simulink model "PID1_kalman"  (Simulink 8.5)
settings: Solver=ode45  StartTime=0.0  StopTime=10  RelTol=1e-3
values from neighbouring files (symbols this model uses):
  arm_home = [ -0.1106   -1.9490   -0.1920    3.1840 ]    [NEW_PID_4DOF.m]    (also in SetPoint_Control.m = [ -0.1106   -1.9490   -0.1920    3.1840    0.2825    0.0969 ; Stochastic_coriolis.m = [  -0.1106   -1.9490   -0.1920    3.1840    0.2825    0.0969; Untitled4.m = [ -0.1106   -1.9490   -0.1920    3.1840    0.2825    0.0969 )
undefined symbols (not defined in the file or in its folder): arm_j2mt, arm_m2jp, bit, CAN_init, enc_per_rev, FT_init, get, hot, MT_init, puck_I_per_Nm, sample_time, Standard, VL1_init, VL2_init
libraries: slrtlib x11, simulink x8, slrtsoftinglib x7, dspadpt3 x7, xpcutilitieslib x4, dspsnks4 x1
settings Model: xpc_rtwmakecfg_data=_xpccanac2pci_  Creator=paulghanem  LastModifiedBy=User  SimulationMode=external  ExtModeTrigDuration=50000
settings SolverCC: EnableConcurrentExecution=on
settings DataIOCC: LimitDataPoints=off  MaxDataPoints=5000000  SaveFormat=Dataset  SignalLoggingSaveFormat=Dataset  SaveOutput=off  InspectSignalLogs=on  SaveTime=off  ReturnWorkspaceOutputs=on
settings OptimizationCC: BlockReduction=off  OptimizeBlockIOStorage=off  BufferReuse=off  GlobalBufferReuse=off  ExpressionFolding=off  ExpressionDepthLimit=128  LocalBlockOutputs=off
settings DebuggingCC: UnderspecifiedInitializationDetection=Simplified  MergeDetectMultiDrivingBlocksExec=error  FcnCallInpInsideContextMsg=EnableAllAsError  StateNameClashWarn=none
settings HardwareCC: ProdIntDivRoundTo=Zero  ProdEndianess=LittleEndian  ProdLongLongMode=on  ProdHWDeviceType=Generic->32-bit x86 compatible
settings RTWCC: SystemTargetFile=slrt.tlc  TemplateMakefile=slrt_default_tmf  Description=Simulink Real-Time  RTWVerbose=off
settings SimulinkRealTimeCC: xPCisModelTimeout=off  xPCModelTimeoutSecs=15
settings ConfigComp: CovMetricSettings=dw  CovHtmlReporting=on  CovSaveCumulativeToWorkspaceVar=on  CovSaveSingleToWorkspaceVar=on  CovExternalEMLEnable=off

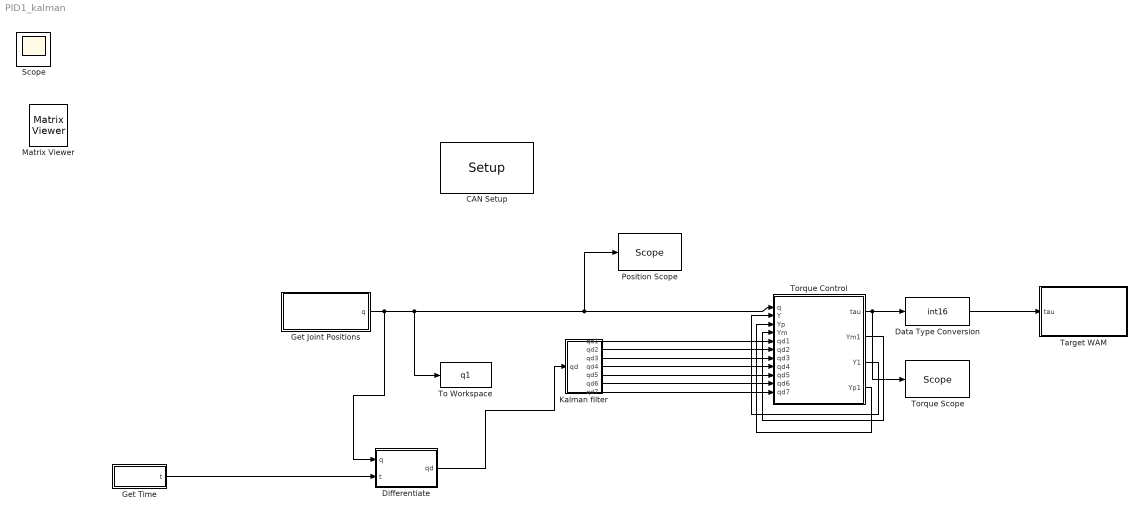
== system PID1_kalman ==
  "CAN Setup " : slrtsoftinglib/CAN-AC2-PCI SJA 1000/Setup   board=1  can1bus=Highspeed (ISO 11898)  can1Baudrate=1 MBaud  can1UserBR=[1,1,4,3]  can2bus=Highspeed (ISO 11898)  can2Baudrate=1 MBaud  can2UserBR=[1,1,4,3]  init=[VL1_init,VL2_init,CAN_init,FT_init,MT_init]  term=[]  bus_off_out=off  bus_off_rec=Off  ioBaseAddress=-1
  Data Type Conversion : DataTypeConversion  OutDataTypeStr=int16
  Differentiate : Subsystem
  Get Joint Positions : Subsystem
  Get Time : Subsystem
  Kalman filter : Subsystem
  Position Scope : slrtlib/Displays and Logging/Scope   scopeno=2  scopetype=Target  autostart=on  viewmode=Numerical  formatstr=['joint_1 %13.8f rad,joint_2 %13.8f rad,joint_3 %13.8f rad,joint_4 %13.8f rad,joint_5 %13.8f rad,joint_6 %13.8f rad,joint_7 %13.8f rad']  grid=on  ylimits=[0,0]  nosamples=1/(10*sample_time)  noprepostsamples=0  interleave=1  triggermode=FreeRun  triggersignal=1  trigsignalfromport=off  triggerlevel=0.0  triggerslope=Either  triggerscope=1  triggersample=0  filename=data.dat  mode=Lazy  writesize=512  autorestart=off  dynamicfilemode=off  maxwritefilesize=512*1024^2
  Target WAM : Subsystem
  To Workspace : ToWorkspace  VariableName=q1  SaveFormat=Structure With Time  SampleTime=-1
  Torque Control : Subsystem
  Torque Scope : slrtlib/Displays and Logging/Scope   scopeno=1  scopetype=Target  autostart=on  viewmode=Numerical  formatstr=['joint_1 %10.5f N-m,joint_2 %10.5f N-m,joint_3 %10.5f N-m,joint_4 %10.5f N-m,joint_5 %10.5f N-m,joint_6 %10.5f N-m,joint_7 %10.5f N-m']  grid=on  ylimits=[0,0]  nosamples=1/(10*sample_time)  noprepostsamples=0  interleave=1  triggermode=FreeRun  triggersignal=1  trigsignalfromport=off  triggerlevel=0.0  triggerslope=Either  triggerscope=1  triggersample=0  filename=data.dat  mode=Lazy  writesize=512  autorestart=off  dynamicfilemode=off  maxwritefilesize=512*1024^2
  Matrix Viewer : dspsnks4/Matrix Viewer  IOType=viewer  ImageParams=off  CMapStr=hot(256)  AxisColorbar=on  AxisParams=off  AxisOrigin=Upper left corner  XLabel=X-axis  YLabel=Y-axis  ZLabel=Z-axis  FigPos=get(0,'defaultfigureposition')  AxisZoom=off
      settings: YMin=-2  YMax=0
  Scope : Scope
  wires:
  Torque Control/1(tau) -> Data Type Conversion/1, Torque Scope/1
  Get Joint Positions/1(q) -> Differentiate/1(q), To Workspace/1, Torque Control/1(q), Position Scope/1
  Data Type Conversion/1 -> Target WAM/1(tau)
  Torque Control/2(Ym1) -> Torque Control/4(Ym)
  Torque Control/3(Y1) -> Torque Control/2(Y)
  Torque Control/4(Yp1) -> Torque Control/3(Yp)
  Differentiate/1(qd) -> Kalman filter/1(qd)
  Get Time/1(t) -> Differentiate/2(t)
  Kalman filter/1(qd1) -> Torque Control/5(qd1)
  Kalman filter/2(qd2) -> Torque Control/6(qd2)
  Kalman filter/3(qd3) -> Torque Control/7(qd3)
  Kalman filter/4(qd4) -> Torque Control/8(qd4)
  Kalman filter/5(qd5) -> Torque Control/9(qd5)
  Kalman filter/6(qd6) -> Torque Control/10(qd6)
  Kalman filter/7(qd7) -> Torque Control/11(qd7)

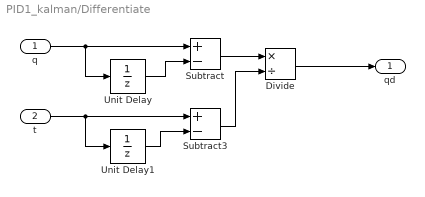
== system PID1_kalman/Differentiate ==
  q : Inport
  t : Inport  Port=2
  Divide : Product  Inputs=*/
  Subtract : Sum  Inputs=+-
  Subtract3 : Sum  Inputs=+-
  Unit Delay : UnitDelay  SampleTime=-1
  Unit Delay1 : UnitDelay  SampleTime=-1
  qd : Outport
  wires:
  q/1 -> Subtract/1, Unit Delay/1
  t/1 -> Unit Delay1/1, Subtract3/1
  Unit Delay1/1 -> Subtract3/2
  Unit Delay/1 -> Subtract/2
  Subtract/1 -> Divide/1
  Divide/1 -> qd/1
  Subtract3/1 -> Divide/2

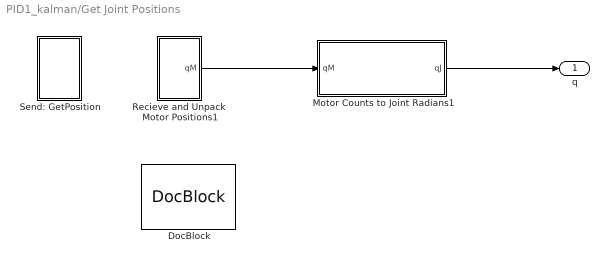
== system PID1_kalman/Get Joint Positions ==
  DocBlock : simulink/Model-Wide Utilities/DocBlock  DocumentType=Text
  Motor Counts to Joint Radians1 : Subsystem
  Recieve and Unpack  Motor Positions1 : Subsystem
  Send: GetPosition : Subsystem
  q : Outport
  wires:
  Motor Counts to Joint Radians1/1(qJ) -> q/1
  Recieve and Unpack  Motor Positions1/1(qM) -> Motor Counts to Joint Radians1/1(qM)

== system PID1_kalman/Get Time ==
  Clock Frequency : Constant  Value=1.193e6
  Divide1 : Product  Inputs=*/
  "xPC Target  Time " : slrtlib/Target Management/Target Information/Session Time   ts=sample_time
  t : Outport
  wires:
  "xPC Target  Time "/1 -> Divide1/1
  Clock Frequency/1 -> Divide1/2
  Divide1/1 -> t/1

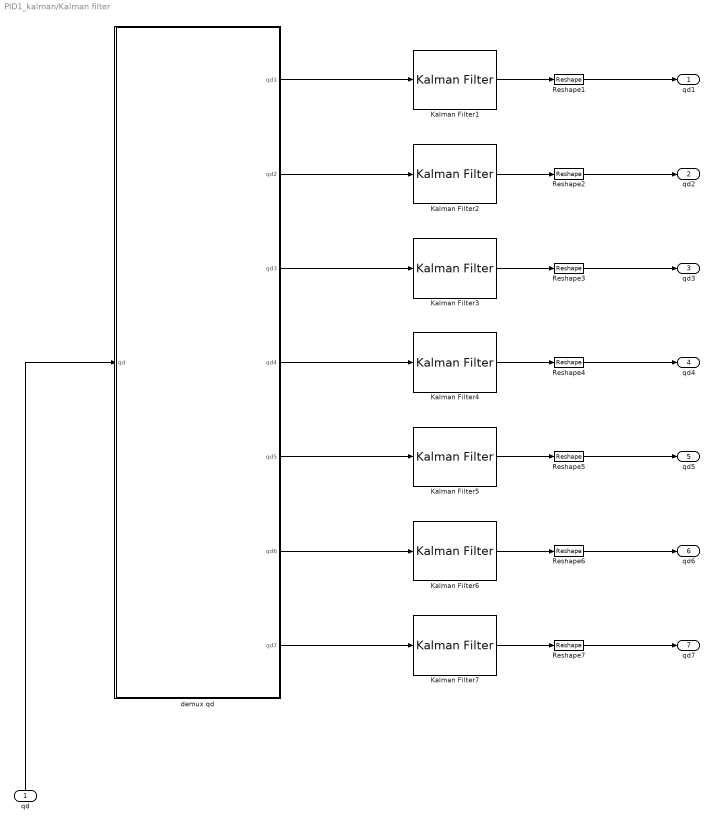
== system PID1_kalman/Kalman filter ==
  qd : Inport
  Kalman Filter1 : dspadpt3/Kalman Filter  num_targets=1  sourceEnable=Always  isReset=off  X=[-0.1106; 0]  P=[1e-4 0 ; 0 1]  A=[1 0.002 ; 0 1]  sourceMeasure=Specify via Dialog  H=[1 0]  Q=[0 0.000 ;0.000 0.004]  R=1e-3  isOutputEstMeasure=on  isOutputEstState=off  isOutputEstError=off  isOutputPrdMeasure=off  isOutputPrdState=off  isOutputPrdError=off
  Kalman Filter2 : dspadpt3/Kalman Filter  num_targets=1  sourceEnable=Always  isReset=on  X=[-1.94900000000000; 0]  P=[1e-4 0 ; 0 1]  A=[1 0.002 ; 0 1]  sourceMeasure=Specify via Dialog  H=[1 0]  Q=[0 0; 0 0.004]  R=5e-2  isOutputEstMeasure=on  isOutputEstState=off  isOutputEstError=off  isOutputPrdMeasure=off  isOutputPrdState=off  isOutputPrdError=off
  Kalman Filter3 : dspadpt3/Kalman Filter  num_targets=1  sourceEnable=Always  isReset=on  X=[-0.192000000000000; 0]  P=[1e-4 0 ; 0 1]  A=[1 0.002 ; 0 1]  sourceMeasure=Specify via Dialog  H=[1 0]  Q=[0 0; 0 0.004]  R=1e-3  isOutputEstMeasure=on  isOutputEstState=off  isOutputEstError=off  isOutputPrdMeasure=off  isOutputPrdState=off  isOutputPrdError=off
  Kalman Filter4 : dspadpt3/Kalman Filter  num_targets=1  sourceEnable=Always  isReset=on  X=[3.18400000000000; 0]  P=[1e-4 0 ; 0 1]  A=[1 0.002 ; 0 1]  sourceMeasure=Specify via Dialog  H=[1 0]  Q=[0 0; 0 0.004]  R=1e-3  isOutputEstMeasure=on  isOutputEstState=off  isOutputEstError=off  isOutputPrdMeasure=off  isOutputPrdState=off  isOutputPrdError=off
  Kalman Filter5 : dspadpt3/Kalman Filter  num_targets=1  sourceEnable=Always  isReset=on  X=[0.282500000000000; 0]  P=[1e-4 0 ; 0 1]  A=[1 0.002 ; 0 1]  sourceMeasure=Specify via Dialog  H=[1 0]  Q=[0 0; 0 0.004]  R=1e-6  isOutputEstMeasure=on  isOutputEstState=off  isOutputEstError=off  isOutputPrdMeasure=off  isOutputPrdState=off  isOutputPrdError=off
  Kalman Filter6 : dspadpt3/Kalman Filter  num_targets=1  sourceEnable=Always  isReset=on  X=[0.0969000000000000; 0]  P=[1e-4 0 ; 0 1]  A=[1 0.002 ; 0 1]  sourceMeasure=Specify via Dialog  H=[1 0]  Q=[0 0; 0 0.004]  R=1e-6  isOutputEstMeasure=on  isOutputEstState=off  isOutputEstError=off  isOutputPrdMeasure=off  isOutputPrdState=off  isOutputPrdError=off
  Kalman Filter7 : dspadpt3/Kalman Filter  num_targets=1  sourceEnable=Always  isReset=on  X=[-0.279800000000000; 0]  P=[1e-4 0 ; 0 1]  A=[1 0.002 ; 0 1]  sourceMeasure=Specify via Dialog  H=[1 0]  Q=[0 0; 0 0.004]  R=1e-6  isOutputEstMeasure=on  isOutputEstState=off  isOutputEstError=off  isOutputPrdMeasure=off  isOutputPrdState=off  isOutputPrdError=off
  Reshape{1..7} (7 alike) : Reshape
  demux qd : Subsystem
  qd1 : Outport
  qd2 : Outport  Port=2
  qd3 : Outport  Port=3
  qd4 : Outport  Port=4
  qd5 : Outport  Port=5
  qd6 : Outport  Port=6
  qd7 : Outport  Port=7
  wires:
  Reshape7/1 -> qd7/1
  Kalman Filter7/1 -> Reshape7/1
  qd/1 -> demux qd/1(qd)
  demux qd/7(qd7) -> Kalman Filter7/1
  demux qd/4(qd4) -> Kalman Filter4/1
  Kalman Filter5/1 -> Reshape5/1
  Reshape5/1 -> qd5/1
  demux qd/5(qd5) -> Kalman Filter5/1
  demux qd/2(qd2) -> Kalman Filter2/1
  demux qd/3(qd3) -> Kalman Filter3/1
  Kalman Filter3/1 -> Reshape3/1
  Kalman Filter2/1 -> Reshape2/1
  Reshape3/1 -> qd3/1
  Reshape2/1 -> qd2/1
  demux qd/6(qd6) -> Kalman Filter6/1
  Reshape6/1 -> qd6/1
  Kalman Filter6/1 -> Reshape6/1
  Kalman Filter4/1 -> Reshape4/1
  Reshape4/1 -> qd4/1
  Reshape1/1 -> qd1/1
  Kalman Filter1/1 -> Reshape1/1
  demux qd/1(qd1) -> Kalman Filter1/1

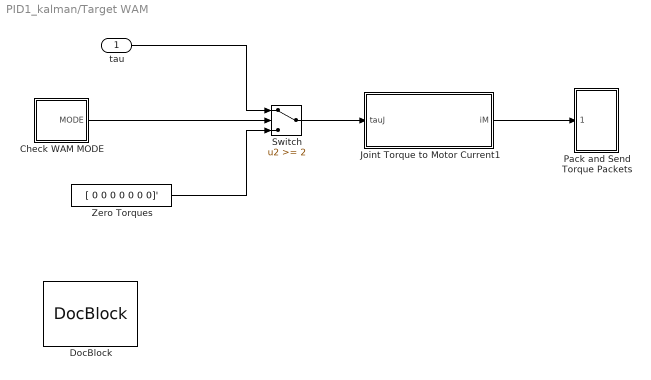
== system PID1_kalman/Target WAM ==
  tau : Inport
  Check WAM MODE : Subsystem
  DocBlock : simulink/Model-Wide Utilities/DocBlock  DocumentType=Text
      content=|
      | This block does all of the communication with the WAM over the CAN card.
      | First we check the WAM mode to see if it in is Shift-Idle or Shift-Active
      | mode. It is necessary to pass this as output, so that PID knows whether it
      | should be integrating on the error or not. If we are in Shift-Idle mode,
      | we send zero torques. Also in this block, we convert joint torque to motor
      | current using the transformations in the documentation. Then we pack the
      | torque packets into a CAN message and send it.
      |
      | To receive joint positions we also send a CAN message which will respond
      | back with the appropriate information. Once we receive the joint positions,
      | we need to differentiate it to get joint velocities (since the WAM does not
      | have tachometers). Finally, passing it through a moving average of the last
      | n readings removes some of the noise and gives us a smoother velocity
      | signal.
  Joint Torque to Motor Current1 : Subsystem
  Pack and Send Torque Packets : Subsystem
  Switch : Switch  Threshold=2
  Zero Torques : Constant  Value=[ 0 0 0 0 0 0 0]'  OutDataTypeStr=int16
  wires:
  Joint Torque to Motor Current1/1(iM) -> Pack and Send Torque Packets/1(Current)
  Switch/1 -> Joint Torque to Motor Current1/1(tauJ)
  tau/1 -> Switch/1
  Zero Torques/1 -> Switch/3
  Check WAM MODE/1(MODE) -> Switch/2

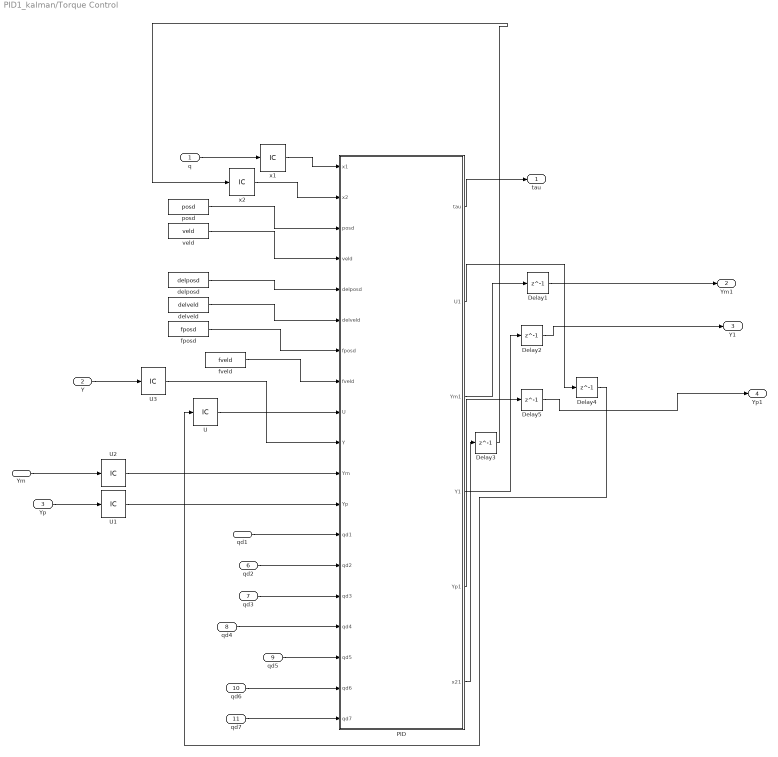
== system PID1_kalman/Torque Control ==
  q : Inport
  Y : Inport  Port=2  PortDimensions=[14]
  Yp : Inport  Port=3  PortDimensions=[14]
  Ym : Inport  Port=4  PortDimensions=[14]
  qd1 : Inport  Port=5
  qd2 : Inport  Port=6
  qd3 : Inport  Port=7
  qd4 : Inport  Port=8
  qd5 : Inport  Port=9
  qd6 : Inport  Port=10
  qd7 : Inport  Port=11
  Delay{1..5} (5 alike) : Delay  DelayLength=1  InitialCondition=0
  PID : MATLAB Function  TreatAsAtomicUnit=on
  U : InitialCondition  Value=[0 0 0 0 0 0 0]
  U1 : InitialCondition  Value="[-0.118379466216232\t-1.94549765955054\t-0.0293926790562203\t3.12033974637458\t0.240671515435818\t-0.0680676596254651\t-0.117976842537181 0 0 0 0 0 0 0]"
  U2 : InitialCondition  Value="[-0.118379466216232\t-1.94549765955054\t-0.0293926790562203\t3.12033974637458\t0.240671515435818\t-0.0680676596254651\t-0.117976842537181 0 0 0 0 0 0 0]"
  U3 : InitialCondition  Value=[-0.118379466216232 -1.94549765955054 -0.0293926790562203 3.12033974637458 0.240671515435818 -0.068067659625465 -0.117976842537181 0 0 0 0 0 0 0]
  "delposd " : FromWorkspace  VariableName=delposd  SampleTime=sample_time
  delveld : FromWorkspace  VariableName=delveld  SampleTime=sample_time
  "fposd " : FromWorkspace  VariableName=fposd  SampleTime=sample_time
  fveld : FromWorkspace  VariableName=fveld  SampleTime=sample_time
  "posd " : FromWorkspace  VariableName=posd  SampleTime=sample_time
  veld : FromWorkspace  VariableName=veld  SampleTime=sample_time
  x1 : InitialCondition  Value="[-0.118379466216232\t-1.94549765955054\t-0.0293926790562203\t3.12033974637458\t0.240671515435818\t-0.0680676596254651\t-0.117976842537181]"
  x2 : InitialCondition  Value=[0 0 0 0 0 0 0]
  tau : Outport
  Ym1 : Outport  Port=2  PortDimensions=[14]
  Y1 : Outport  Port=3  PortDimensions=[14]
  Yp1 : Outport  Port=4  PortDimensions=[14]
  wires:
  PID/1(tau) -> tau/1
  q/1 -> x1/1
  x1/1 -> PID/1(x1)
  PID/6(x21) -> Delay3/1
  Delay3/1 -> x2/1
  PID/2(U1) -> Delay4/1
  Delay4/1 -> U/1
  U/1 -> PID/9(U)
  x2/1 -> PID/2(x2)
  "posd "/1 -> PID/3(posd)
  veld/1 -> PID/4(veld)
  "delposd "/1 -> PID/5(delposd)
  delveld/1 -> PID/6(delveld)
  "fposd "/1 -> PID/7(fposd)
  fveld/1 -> PID/8(fveld)
  PID/3(Ym1) -> Delay1/1
  PID/4(Y1) -> Delay2/1
  PID/5(Yp1) -> Delay5/1
  Delay1/1 -> Ym1/1
  Delay2/1 -> Y1/1
  Delay5/1 -> Yp1/1
  Y/1 -> U3/1
  Ym/1 -> U2/1
  Yp/1 -> U1/1
  U3/1 -> PID/10(Y)
  U2/1 -> PID/11(Ym)
  U1/1 -> PID/12(Yp)
  qd1/1 -> PID/13(qd1)
  qd3/1 -> PID/15(qd3)
  qd5/1 -> PID/17(qd5)
  qd2/1 -> PID/14(qd2)
  qd4/1 -> PID/16(qd4)
  qd6/1 -> PID/18(qd6)
  qd7/1 -> PID/19(qd7)

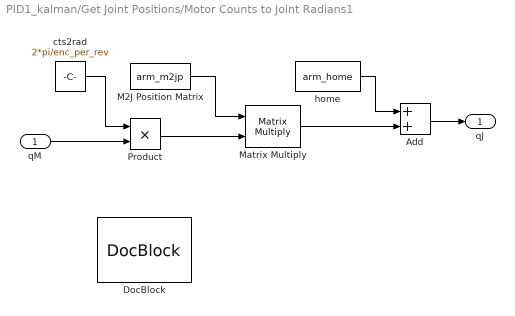
== system PID1_kalman/Get Joint Positions/Motor Counts to Joint Radians1 ==
  qM : Inport
  Add : Sum
  DocBlock : simulink/Model-Wide Utilities/DocBlock  DocumentType=Text
      content=|
      | Here we do the simple conversion from motor position to joint position,
      | then convert encoder counts to joint radians, then account for the offset
      | in the home position to finally output the joint position in radians. The
      | M2J position matrix can be found in the documentation. Joint 4 has a -18 as
      | opposed to +18 because the motor was reversed at one point during a repair.
      | I believe newer models of the WAM adhere to this -18.
  M2J Position Matrix : Constant  Value=arm_m2jp
  Matrix Multiply : Product  Multiplication=Matrix(*)
  Product : Product  OutMin=[-8192]  OutMax=[8191]  RndMeth=Zero
  cts2rad : Constant  Value=2*pi/enc_per_rev
  home : Constant  Value=arm_home
  qJ : Outport
  wires:
  qM/1 -> Product/2
  Add/1 -> qJ/1
  Matrix Multiply/1 -> Add/2
  home/1 -> Add/1
  cts2rad/1 -> Product/1
  M2J Position Matrix/1 -> Matrix Multiply/1
  Product/1 -> Matrix Multiply/2

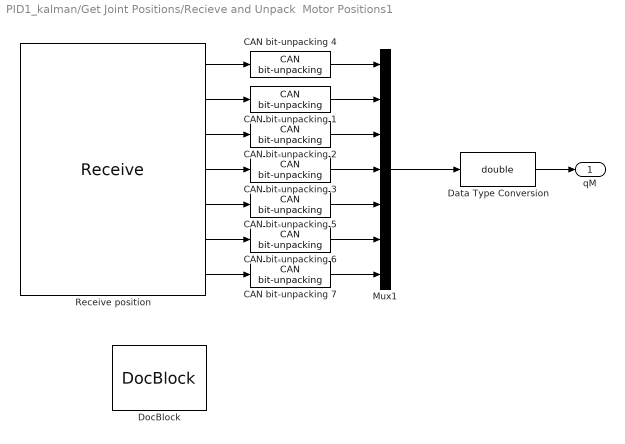
== system PID1_kalman/Get Joint Positions/Recieve and Unpack  Motor Positions1 ==
  CAN bit-unpacking {1..7} (7 alike) : slrtlib/CAN/Utilities/CAN bit-unpacking   bitpatterns={ [16:23, 8:15, 0:5,-1, -1] }  dtypes={ 'int32'}
  Data Type Conversion : DataTypeConversion  OutDataTypeStr=double
  DocBlock : simulink/Model-Wide Utilities/DocBlock  DocumentType=Text
  Mux1 : Mux  Inputs=7
  "Receive position " : slrtsoftinglib/CAN-AC2-PCI SJA 1000/Receive   board=1  canPort=CAN 1  range=Standard (11-bit)  ids=[bin2dec('10000100011'),bin2dec('10001000011'),bin2dec('10001100011'),bin2dec('10010000011'),bin2dec('10010100011'),bin2dec('10011000011'),bin2dec('10011100011')]  lengths=0  output=Data  inten=on  ts=sample_time  ididx=[0,1,2,3,5,6,7]
  qM : Outport
  wires:
  Mux1/1 -> Data Type Conversion/1
  "Receive position "/1 -> CAN bit-unpacking 4/1
  "Receive position "/2 -> CAN bit-unpacking 1/1
  "Receive position "/3 -> CAN bit-unpacking 2/1
  "Receive position "/4 -> CAN bit-unpacking 3/1
  CAN bit-unpacking 4/1 -> Mux1/1
  CAN bit-unpacking 1/1 -> Mux1/2
  CAN bit-unpacking 2/1 -> Mux1/3
  CAN bit-unpacking 3/1 -> Mux1/4
  Data Type Conversion/1 -> qM/1
  "Receive position "/5 -> CAN bit-unpacking 5/1
  "Receive position "/6 -> CAN bit-unpacking 6/1
  "Receive position "/7 -> CAN bit-unpacking 7/1
  CAN bit-unpacking 5/1 -> Mux1/5
  CAN bit-unpacking 6/1 -> Mux1/6
  CAN bit-unpacking 7/1 -> Mux1/7

== system PID1_kalman/Get Joint Positions/Send: GetPosition ==
  Bit Packing : xpcutilitieslib/Bit Packing   MaskBitPatterns={[0:7]}  MaskPackDataType=double  MaskPackDataSize=[1]
  DocBlock : simulink/Model-Wide Utilities/DocBlock  DocumentType=Text
  Send to all motors : slrtsoftinglib/CAN-AC2-PCI SJA 1000/Send   board=1  canPort=CAN 1  range=Standard (11-bit)  ids=1024  sizes=[1]  output=off  ts=sample_time  ididx=[2]
  get position : Constant  Value=[48]  OutDataTypeStr=int8
  wires:
  Bit Packing/1 -> Send to all motors/1
  get position/1 -> Bit Packing/1

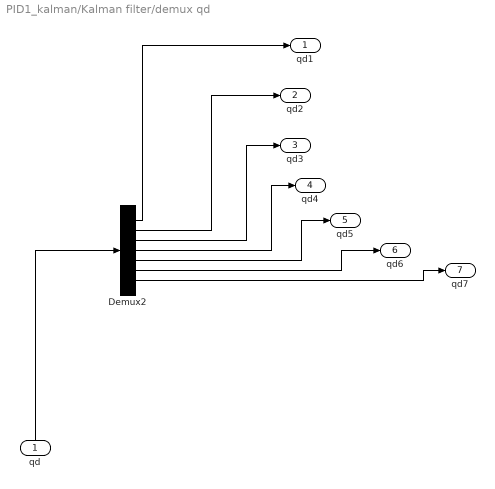
== system PID1_kalman/Kalman filter/demux qd ==
  qd : Inport
  Demux2 : Demux  Outputs=7
  qd1 : Outport
  qd2 : Outport  Port=2
  qd3 : Outport  Port=3
  qd4 : Outport  Port=4
  qd5 : Outport  Port=5
  qd6 : Outport  Port=6
  qd7 : Outport  Port=7
  wires:
  qd/1 -> Demux2/1
  Demux2/1 -> qd1/1
  Demux2/2 -> qd2/1
  Demux2/3 -> qd3/1
  Demux2/4 -> qd4/1
  Demux2/5 -> qd5/1
  Demux2/6 -> qd6/1
  Demux2/7 -> qd7/1

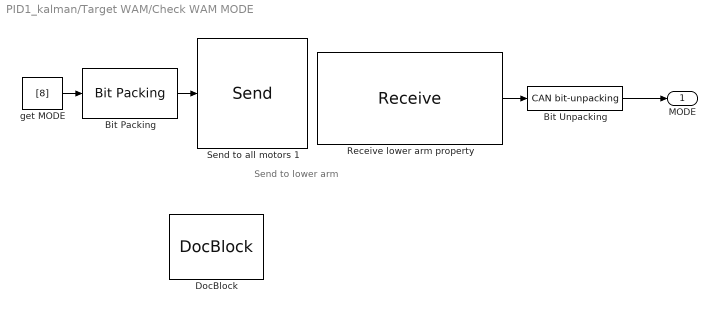
== system PID1_kalman/Target WAM/Check WAM MODE ==
  note: Send to lower arm
  "Bit Packing " : xpcutilitieslib/Bit Packing   MaskBitPatterns={[0:7]}  MaskPackDataType=double  MaskPackDataSize=[1]
  Bit Unpacking : slrtlib/CAN/Utilities/CAN bit-unpacking   bitpatterns={[16:31]}  dtypes={ 'int16'}
  DocBlock : simulink/Model-Wide Utilities/DocBlock  DocumentType=Text
      content=|
      | Here we send an 8 to the lower arm. Property 8 is the MODE and the
      | 1028 (1 00000 00100) means to "set a lower arm property". Finally we
      | receive the mode property from CAN ID 1158, then do some bit unpacking.
      | All of this is well documentated in the "CAN Communication Spec" of the
      | Barrett documentation.
  Receive lower arm property : slrtsoftinglib/CAN-AC2-PCI SJA 1000/Receive   board=1  canPort=CAN 1  range=Standard (11-bit)  ids=[bin2dec('10010000110')]  lengths=0  output=Data  inten=on  ts=sample_time  ididx=[4]
  Send to all motors 1 : slrtsoftinglib/CAN-AC2-PCI SJA 1000/Send   board=1  canPort=CAN 1  range=Standard (11-bit)  ids=[1028]  sizes=[1]  output=off  ts=sample_time  ididx=[5]
  get MODE : Constant  Value=[8]  OutDataTypeStr=uint8
  MODE : Outport
  wires:
  "Bit Packing "/1 -> Send to all motors 1/1
  Receive lower arm property/1 -> Bit Unpacking/1
  get MODE/1 -> "Bit Packing "/1
  Bit Unpacking/1 -> MODE/1

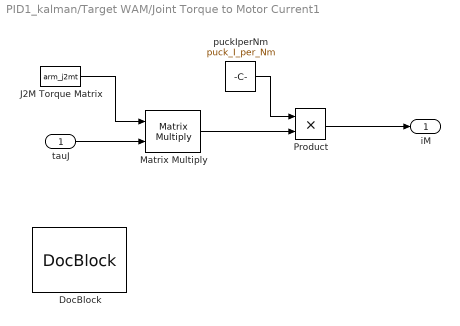
== system PID1_kalman/Target WAM/Joint Torque to Motor Current1 ==
  tauJ : Inport
  DocBlock : simulink/Model-Wide Utilities/DocBlock  DocumentType=Text
  J2M Torque Matrix : Constant  Value=arm_j2mt
  Matrix Multiply : Product  Multiplication=Matrix(*)
  Product : Product  RndMeth=Zero
  puckIperNm : Constant  Value=puck_I_per_Nm
  iM : Outport
  wires:
  J2M Torque Matrix/1 -> Matrix Multiply/1
  Matrix Multiply/1 -> Product/2
  puckIperNm/1 -> Product/1
  Product/1 -> iM/1
  tauJ/1 -> Matrix Multiply/2

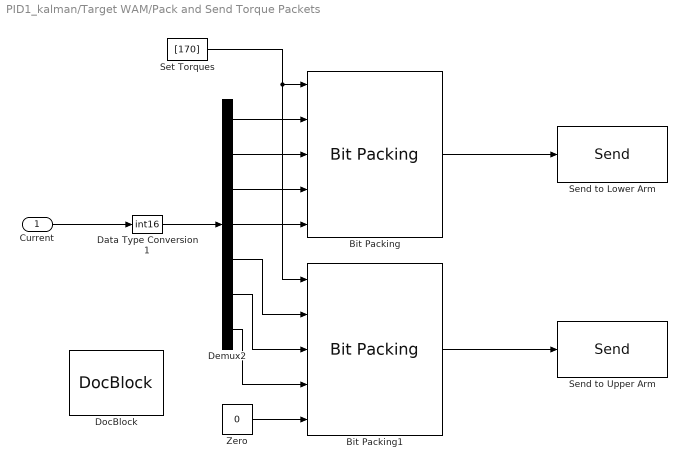
== system PID1_kalman/Target WAM/Pack and Send Torque Packets ==
  Current : Inport
  Bit Packing : xpcutilitieslib/Bit Packing   MaskBitPatterns={[0:7] [18:23 8:15] [36:39 24:31 16:17] [54:55 40:47 32:35] [56:63 48:53]}  MaskPackDataType=double  MaskPackDataSize=[1]
  Bit Packing1 : xpcutilitieslib/Bit Packing   MaskBitPatterns={[0:7] [18:23 8:15] [36:39 24:31 16:17] [54:55 40:47 32:35] [56:63 48:53]}  MaskPackDataType=double  MaskPackDataSize=[1]
  Data Type Conversion1 : DataTypeConversion  OutMin=[-8191]  OutMax=[8191]  OutDataTypeStr=int16  RndMeth=Zero
  Demux2 : Demux  Outputs=7
  DocBlock : simulink/Model-Wide Utilities/DocBlock  DocumentType=Text
  Send to Lower Arm : slrtsoftinglib/CAN-AC2-PCI SJA 1000/Send   board=1  canPort=CAN 1  range=Standard (11-bit)  ids=bin2dec('10000000001')  sizes=[8]  output=off  ts=sample_time  ididx=[3]
  Send to Upper Arm : slrtsoftinglib/CAN-AC2-PCI SJA 1000/Send   board=1  canPort=CAN 1  range=Standard (11-bit)  ids=bin2dec('10000000010')  sizes=[8]  output=off  ts=sample_time  ididx=[4]
  "Set Torques " : Constant  Value=[170]  OutDataTypeStr=uint8
  Zero : Constant  Value=0  OutDataTypeStr=int16
  wires:
  "Set Torques "/1 -> Bit Packing/1, Bit Packing1/1
  Bit Packing/1 -> Send to Lower Arm/1
  Demux2/1 -> Bit Packing/2
  Demux2/2 -> Bit Packing/3
  Demux2/3 -> Bit Packing/4
  Demux2/4 -> Bit Packing/5
  Current/1 -> Data Type Conversion1/1
  Data Type Conversion1/1 -> Demux2/1
  Bit Packing1/1 -> Send to Upper Arm/1
  Demux2/5 -> Bit Packing1/2
  Demux2/6 -> Bit Packing1/3
  Demux2/7 -> Bit Packing1/4
  Zero/1 -> Bit Packing1/5

== matlab function Torque Control/PID ==
  data: x1 input double; x2 input double; posd input double; tau output double; veld input double; delposd input double; delveld input double; fposd input double; fveld input double; U input double; U1 output double; Ym1 output double; Y1 output double; Yp1 output double; x21 output double; Y input double; Ym input double; Yp input double; qd1 input double; qd2 input double; qd3 input double; qd4 input double; qd5 input double; qd6 input double; qd7 input double
%
% gravComp7DOFNum Compute inverse dynamics via recursive Newton-Euler formulation
%
% Recursive Newton-Euler for standard Denavit-Hartenberg notation.
%

% Copyright (C) 1993-2011, by Peter I. Corke
%
% This file originally was part of The Robotics Toolbox for Matlab (RTB).
%
% http://www.petercorke.com

%
% Simplified from rne_dh for 7DOF WAM to compute only torque from gravity by Hans Vorsteveld
% Does not use structures from RTB, only the RNE algorithm
%

function [tau,U1,Ym1,Y1,Yp1,x21] = PID(x1,x2,posd,veld,delposd,delveld,fposd,fveld,U,Y,Ym,Yp,qd1,qd2,qd3,qd4,qd5,qd6,qd7)

%-------------------------------------------------------------------------------------
%   SETUP THE ARM
%-------------------------------------------------------------------------------------    
    n = 14;p = 7; q = 14;
    
 Ts=0.002; 


 


yddel=[delposd;delveld];
yd = [posd;veld];
fyd=[fposd;fveld];


 

%initial conditions
%x1 = [-0.11060;-1.949;-0.1920;3.1840;0.2825;0.09690;-0.27980];
%x2 = zeros(7,1);
%U = zeros(7,1);
Ae = (1-Ts)*eye(n);
C= eye(14);
Ce = C;
Iq = eye(q);
Oq = zeros(q);
H = [Iq Oq Oq -Ce*Ae;Iq Oq Oq zeros(q,n);Oq Iq Oq zeros(q,n);zeros(n,q) zeros(n,q) zeros(n,q) Ae];
Ib = zeros(3*q,3*q+n);
for k11 = 1:3*q,Ib(k11,k11) = 1;end
sig = 1e-4;
sigR = sig;
sigQ = 1e-3;
P = 1e-8*eye(3*q+n);
Rb = (sigR^2)*diag(1*ones(3*q,1));
Q = sigQ^2*eye(n);





 Be = Ts*[zeros(7,7);inv(D(x1))];
    Delyd=[fyd-yd];
    Del2yd = Delyd*Delyd';
   
    Gd = [Del2yd Oq Oq zeros(q,n); Oq Oq Oq zeros(q,n); Oq Oq Oq zeros(q,n);zeros(n,q) zeros(n,q) zeros(n,q) Q];
   
    
    
    EE = [Ce*Be;zeros(q,p);zeros(q,p);-Be];
    K = inv(EE'*EE)*EE'*H*P*Ib'*inv(Ib*P*Ib' + Rb);
    PHI = H - EE*K*Ib;

     P = PHI*P*PHI' + EE*K*Rb*K'*EE' + Gd;
    K1 = K(:,1:q);
    K2 = K(:,q+1:2*q);
    K3 = K(:,2*q+1:3*q);
    
    
      %  E = yd - Y ;
       % Ep = ydfut-Yp ;
        %U = U + K1*Ep + K2*E;
        %Ym = Y;
        %Y = Yp;
         %x_1 = x1 ;
       
         %x_11 = x_1; %Since at t=0, velocity is zero
        %XX2 = zeros(7,1);
        %x_22= (-inv(D(x_1))*(transpose(G(x_1)))+ inv(D(x_1))*U)*Ts + XX2 ;
        %Yp = [x_11' x_22']';
       
    
        Em = yddel - Ym ;
        E = yd - Y ;
        Ep = fyd-Yp ;
        U = U + K1*Ep + K2*E + K3*Em;
        Ym = Y;
        Y = Yp;
        
        x_1 = x1;
        
         %
        pos_meas = x1 ; % In experimental work you do not add noise instead you only use measurement of position
        x_11 =  x2*Ts + pos_meas; % Here we are estimating position using the extimate of x2 and measurement of x1 at present time
        
       % XX2 = (x_11-x_1)/Ts; %
       XX2=[qd1;qd2;qd3;qd4;qd5;qd6;qd7];
       
        x_22= (-inv(D(pos_meas))*((G(pos_meas)))+ inv(D(pos_meas))*U)*Ts + XX2 ;
       
       
        
        Yp = [x_11' x_22']';
        tau=U;
        Yp1=Yp;
        Ym1=Ym;
        Y1=Y;
        U1=U;
        x21= x_22;
    
   
end 

function G = G(q)

DH_a = [0 0 0.045 -0.045 0 0 0];
    DH_d = [0 0 .55 0 0.3 0 0.061];
    DH_alpha = [-pi/2 pi/2 -pi/2 pi/2 -pi/2 pi/2 0];
 
    m = [10.7676 3.87 1.8022 2.4 0.1237 0.4979886 0.07548270];
    
    com = zeros(3,7);
    com(:,1) = [-0.00443422; 0.12189039; -0.00066489];
    com(:,2) = [-0.00236983; 0.03105614; 0.01542114 ];
    com(:,3) = [-0.03825858; 0.20750770; 0.00003309];
    com(:,4) = [ 0.00498512;-0.00022942;0.13271662 ];
    com(:,5) = [0.00008921;0.00511217;0.00435824];
    com(:,6) = [-0.00012262;-0.01703194;0.02468336];
    com(:,7) = [-0.00007974;0.00016313;-0.00323552 ];
     
    
    T = zeros(4,4,7);
     
for j=1:7,
        a = DH_a(j);
        d = DH_d(j);
        alpha = DH_alpha(j);
        T(:,:,j) = getTransformDH(a, d, alpha, q(j));
end 
comstar = zeros(4,7);
    comstar(:,1) = [com(:,1);1];
    comstar(:,2) = [com(:,2);1];
    comstar(:,3) = [com(:,3);1];
    comstar(:,4) = [com(:,4);1];
    comstar(:,5) = [com(:,5);1];
    comstar(:,6) = [com(:,6);1];
    comstar(:,7) = [ com(:,7);1];
  
    Q=[0,-1,0,0;
     1,0,0,0;
     0,0,0,0;
     0,0,0,0];
   
 gravity=[0,0,-9.81,0];
 G=zeros(7,1);
 
   G(1)= -m(1)*gravity*Q*T(:,:,1)*comstar(:,1)-m(2)*gravity*Q*T(:,:,1)*T(:,:,2)*comstar(:,2)-m(3)*gravity*Q*T(:,:,1)*T(:,:,2)*T(:,:,3)*comstar(:,3)-m(4)*gravity*Q*T(:,:,1)*T(:,:,2)*T(:,:,3)*T(:,:,4)*comstar(:,4)-m(5)*gravity*Q*T(:,:,1)*T(:,:,2)*T(:,:,3)*T(:,:,4)*T(:,:,5)*comstar(:,5)-m(6)*gravity*Q*T(:,:,1)*T(:,:,2)*T(:,:,3)*T(:,:,4)*T(:,:,5)*T(:,:,6)*comstar(:,6)-m(7)*gravity*Q*T(:,:,1)*T(:,:,2)*T(:,:,3)*T(:,:,4)*T(:,:,5)*T(:,:,6)*T(:,:,7)*comstar(:,7);   
   G(2)= -m(2)*gravity*T(:,:,1)*Q*T(:,:,2)*comstar(:,2)-m(3)*gravity*T(:,:,1)*Q*T(:,:,2)*T(:,:,3)*comstar(:,3)-m(4)*gravity*T(:,:,1)*Q*T(:,:,2)*T(:,:,3)*T(:,:,4)*comstar(:,4)-m(5)*gravity*T(:,:,1)*Q*T(:,:,2)*T(:,:,3)*T(:,:,4)*T(:,:,5)*comstar(:,5)-m(6)*gravity*T(:,:,1)*Q*T(:,:,2)*T(:,:,3)*T(:,:,4)*T(:,:,5)*T(:,:,6)*comstar(:,6)-m(7)*gravity*T(:,:,1)*Q*T(:,:,2)*T(:,:,3)*T(:,:,4)*T(:,:,5)*T(:,:,6)*T(:,:,7)*comstar(:,7);
   G(3)= -m(3)*gravity*T(:,:,1)*T(:,:,2)*Q*T(:,:,3)*comstar(:,3)-m(4)*gravity*T(:,:,1)*T(:,:,2)*Q*T(:,:,3)*T(:,:,4)*comstar(:,4)-m(5)*gravity*T(:,:,1)*T(:,:,2)*Q*T(:,:,3)*T(:,:,4)*T(:,:,5)*comstar(:,5)-m(6)*gravity*T(:,:,1)*T(:,:,2)*Q*T(:,:,3)*T(:,:,4)*T(:,:,5)*T(:,:,6)*comstar(:,6)-m(7)*gravity*T(:,:,1)*T(:,:,2)*Q*T(:,:,3)*T(:,:,4)*T(:,:,5)*T(:,:,6)*T(:,:,7)*comstar(:,7);
   G(4)= -m(4)*gravity*T(:,:,1)*T(:,:,2)*T(:,:,3)*Q*T(:,:,4)*comstar(:,4)-m(5)*gravity*T(:,:,1)*T(:,:,2)*T(:,:,3)*Q*T(:,:,4)*T(:,:,5)*comstar(:,5)-m(6)*gravity*T(:,:,1)*T(:,:,2)*T(:,:,3)*Q*T(:,:,4)*T(:,:,5)*T(:,:,6)*comstar(:,6)-m(7)*gravity*T(:,:,1)*T(:,:,2)*T(:,:,3)*Q*T(:,:,4)*T(:,:,5)*T(:,:,6)*T(:,:,7)*comstar(:,7);
   G(5)= -m(5)*gravity*T(:,:,1)*T(:,:,2)*T(:,:,3)*T(:,:,4)*Q*T(:,:,5)*comstar(:,5)-m(6)*gravity*T(:,:,1)*T(:,:,2)*T(:,:,3)*T(:,:,4)*Q*T(:,:,5)*T(:,:,6)*comstar(:,6)-m(7)*gravity*T(:,:,1)*T(:,:,2)*T(:,:,3)*T(:,:,4)*Q*T(:,:,5)*T(:,:,6)*T(:,:,7)*comstar(:,7);
   G(6)= -m(6)*gravity*T(:,:,1)*T(:,:,2)*T(:,:,3)*T(:,:,4)*T(:,:,5)*Q*T(:,:,6)*comstar(:,6)-m(7)*gravity*T(:,:,1)*T(:,:,2)*T(:,:,3)*T(:,:,4)*T(:,:,5)*Q*T(:,:,6)*T(:,:,7)*comstar(:,7);
   G(7)= -m(7)*gravity*T(:,:,1)*T(:,:,2)*T(:,:,3)*T(:,:,4)*T(:,:,5)*T(:,:,6)*Q*T(:,:,7)*comstar(:,7);
   
end 
function bq = bq(qd)
 
 
 
s=20;
bc = [2.516; 2.581; 2.038; 0.956; 0.323; 0.315; 0.066];
B =  [1.142; 0.946; 0.309; 0.255; 0.025; 0.039; 0.004];
 
bq = bc.*atan(s*qd)*2/pi+B.*qd;
end 

function D =D(q)
DH_a = [0 0 0.045 -0.045 0 0 0];
    DH_d = [0 0 .55 0 0.3 0 0.061];
    DH_alpha = [-pi/2 pi/2 -pi/2 pi/2 -pi/2 pi/2 0];
 
    m = [10.7676 3.87 1.8022 2.4 0.1237 0.4179886 0.07548270];
    
     
    
    com = zeros(3,7);
   com(:,1) = [-0.00443422; 0.12189039; -0.00066489];
    com(:,2) = [-0.00236983; 0.03105614; 0.01542114 ];
    com(:,3) = [-0.03825858; 0.20750770; 0.00003309];
    com(:,4) = [ 0.00498512;-0.00022942;0.13271662 ];
    com(:,5) = [0.00008921;0.00511217;0.00435824];
    com(:,6) = [-0.00012262;-0.01703194;0.02468336];
    com(:,7) = [-0.00007974;0.00016313;-0.00323552 ];
     
    I=zeros(3,3,7);
    
     I(:,:,1) = [ 0.29486350 , -0.00795023 ,-0.00009311;
                 -0.00795023 , 0.11350017 , -0.00018711;
                -0.00009311 , -0.00018711 , 0.25065343];
    I(:,:,2) =[0.02606840 ,-0.00001346 , -0.00011701;
               -0.00001346,  0.01472202 ,0.00003659;
               -0.00011701 , 0.00003659,  0.01934814];
    I(:,:,3) = [0.13671601,  -0.01680434,  0.00000510;
               -0.01680434 , 0.00588354 , -0.00000530;
                0.00000510 , -0.00000530 , 0.13951371];
    I(:,:,4) = [ 0.05719268 , 0.00001467 , 0.00008193;
                 0.00001467 , 0.05716470 , -0.00009417;
                 0.00008193 , -0.00009417 , 0.00300441] ;
    I(:,:,5) =[0.00005587 , 0.00000026,  0.00000000;
               0.00000026 , 0.00007817,  -0.00000083;
               0.00000000 , -0.00000083,  0.00006594];
    I(:,:,6) = [0.00093106,  0.00000148 , -0.00000201;
                0.00000148,  0.00049833 , -0.00022162;
               -0.00000201,  -0.00022162,  0.00057483];
   I(:,:,7) = [0.00003845,  -0.00000019 , 0.00000002;
                -0.00000019, 0.00003878 , -0.00000004;
                0.00000002 ,  -0.00000004, 0.00007408 ];
            T=zeros(4,4,7);
  
             
for j=1:7,
        a = DH_a(j);
        d = DH_d(j);
        alpha = DH_alpha(j);
        T(:,:,j) = getTransformDH(a, d, alpha, q(j));
end 
 
 
 
 
   comstar = zeros(4,7);
    comstar(:,1) = [com(:,1);1];
    comstar(:,2) = [com(:,2);1];
    comstar(:,3) = [com(:,3);1];
    comstar(:,4) = [com(:,4);1];
    comstar(:,5) = [com(:,5);1];
    comstar(:,6) = [com(:,6);1];
    comstar(:,7) = [ com(:,7);1];
  
    Q=[0,-1,0,0;
     1,0,0,0;
     0,0,0,0;
     0,0,0,0];
   
U=zeros(4,4,7,7);
   U(:,:,1,1)= Q*T(:,:,1);
   U(:,:,2,1)= Q*T(:,:,1)*T(:,:,2);
   U(:,:,3,1)= Q*T(:,:,1)*T(:,:,2)*T(:,:,3);
   U(:,:,4,1)= Q*T(:,:,1)*T(:,:,2)*T(:,:,3)*T(:,:,4);
   U(:,:,5,1)= Q*T(:,:,1)*T(:,:,2)*T(:,:,3)*T(:,:,4)*T(:,:,5);
   U(:,:,6,1)= Q*T(:,:,1)*T(:,:,2)*T(:,:,3)*T(:,:,4)*T(:,:,5)*T(:,:,6);
   U(:,:,7,1)= Q*T(:,:,1)*T(:,:,2)*T(:,:,3)*T(:,:,4)*T(:,:,5)*T(:,:,6)*T(:,:,7);
   
   
   U(:,:,2,2)= T(:,:,1)*Q*T(:,:,2);
   U(:,:,3,2)= T(:,:,1)*Q*T(:,:,2)*T(:,:,3);
   U(:,:,4,2)= T(:,:,1)*Q*T(:,:,2)*T(:,:,3)*T(:,:,4);
   U(:,:,5,2)= T(:,:,1)*Q*T(:,:,2)*T(:,:,3)*T(:,:,4)*T(:,:,5);
   U(:,:,6,2)= T(:,:,1)*Q*T(:,:,2)*T(:,:,3)*T(:,:,4)*T(:,:,5)*T(:,:,6);
   U(:,:,7,2)= T(:,:,1)*Q*T(:,:,2)*T(:,:,3)*T(:,:,4)*T(:,:,5)*T(:,:,6)*T(:,:,7);
   
  
   U(:,:,3,3)= T(:,:,1)*T(:,:,2)*Q*T(:,:,3);
   U(:,:,4,3)= T(:,:,1)*T(:,:,2)*Q*T(:,:,3)*T(:,:,4);
   U(:,:,5,3)= T(:,:,1)*T(:,:,2)*Q*T(:,:,3)*T(:,:,4)*T(:,:,5);
   U(:,:,6,3)= T(:,:,1)*T(:,:,2)*Q*T(:,:,3)*T(:,:,4)*T(:,:,5)*T(:,:,6);
   U(:,:,7,3)= T(:,:,1)*T(:,:,2)*Q*T(:,:,3)*T(:,:,4)*T(:,:,5)*T(:,:,6)*T(:,:,7);
   
   U(:,:,4,4)= T(:,:,1)*T(:,:,2)*T(:,:,3)*Q*T(:,:,4);
   U(:,:,5,4)= T(:,:,1)*T(:,:,2)*T(:,:,3)*Q*T(:,:,4)*T(:,:,5);
   U(:,:,6,4)= T(:,:,1)*T(:,:,2)*T(:,:,3)*Q*T(:,:,4)*T(:,:,5)*T(:,:,6);
   U(:,:,7,4)= T(:,:,1)*T(:,:,2)*T(:,:,3)*Q*T(:,:,4)*T(:,:,5)*T(:,:,6)*T(:,:,7);
   
   U(:,:,5,5)= T(:,:,1)*T(:,:,2)*T(:,:,3)*T(:,:,4)*Q*T(:,:,5);
   U(:,:,6,5)= T(:,:,1)*T(:,:,2)*T(:,:,3)*T(:,:,4)*Q*T(:,:,5)*T(:,:,6);
   U(:,:,7,5)= T(:,:,1)*T(:,:,2)*T(:,:,3)*T(:,:,4)*Q*T(:,:,5)*T(:,:,6)*T(:,:,7);
   
   U(:,:,6,6)= T(:,:,1)*T(:,:,2)*T(:,:,3)*T(:,:,4)*T(:,:,5)*Q*T(:,:,6);
   U(:,:,7,6)= T(:,:,1)*T(:,:,2)*T(:,:,3)*T(:,:,4)*T(:,:,5)*Q*T(:,:,6)*T(:,:,7);
   
   U(:,:,7,7)= T(:,:,1)*T(:,:,2)*T(:,:,3)*T(:,:,4)*T(:,:,5)*T(:,:,6)*Q*T(:,:,7);
   
   
   
  
   J=zeros(4,4,7);
 
   
   J(:,:,1)=[0.5*(-I(1,1,1)+I(2,2,1)+I(3,3,1)), I(1,2,1), I(1,3,1), m(1)*com(1,1);
             I(1,2,1) ,0.5*(I(1,1,1)-I(2,2,1)+I(3,3,1)), I(2,3,1), m(1)*com(2,1);
             I(1,3,1), I(2,3,1), 0.5*(I(1,1,1)+I(2,2,1)-I(3,3,1)), m(1)*com(3,1);
              m(1)*com(1,1), m(1)*com(2,1), m(1)*com(3,1), m(1)];
   
    J(:,:,2)=[0.5*(-I(1,1,2)+I(2,2,2)+I(3,3,2)), I(1,2,2), I(1,3,2), m(2)*com(1,2);
             I(1,2,2) ,0.5*(I(1,1,2)-I(2,2,2)+I(3,3,2)), I(2,3,2), m(2)*com(2,2);
             I(1,3,2), I(2,3,2), 0.5*(I(1,1,2)+I(2,2,2)-I(3,3,2)), m(2)*com(3,2);
              m(2)*com(1,2), m(2)*com(2,2), m(2)*com(3,2), m(2)];
   
          
     J(:,:,3)=[0.5*(-I(1,1,3)+I(2,2,3)+I(3,3,3)), I(1,2,3), I(1,3,3), m(3)*com(1,3);
             I(1,2,3) ,0.5*(I(1,1,3)-I(2,2,3)+I(3,3,3)), I(2,3,3), m(3)*com(2,3);
             I(1,3,3), I(2,3,3), 0.5*(I(1,1,3)+I(2,2,3)-I(3,3,3)), m(3)*com(3,3);
              m(3)*com(1,3), m(3)*com(2,3), m(3)*com(3,3), m(3)];      
   
   
    J(:,:,4)=[0.5*(-I(1,1,4)+I(2,2,4)+I(3,3,4)), I(1,2,4), I(1,3,4), m(4)*com(1,4);
             I(1,2,4) ,0.5*(I(1,1,4)-I(2,2,4)+I(3,3,4)), I(2,3,4), m(4)*com(2,4);
             I(1,3,4), I(2,3,4), 0.5*(I(1,1,4)+I(2,2,4)-I(3,3,4)), m(4)*com(3,4);
              m(4)*com(1,4), m(4)*com(2,4), m(4)*com(3,4), m(4)];
   
   
    J(:,:,5)=[0.5*(-I(1,1,5)+I(2,2,5)+I(3,3,5)), I(1,2,5), I(1,3,5), m(5)*com(1,5);
             I(1,2,5) ,0.5*(I(1,1,5)-I(2,2,5)+I(3,3,5)), I(2,3,5), m(5)*com(2,5);
             I(1,3,5), I(2,3,5), 0.5*(I(1,1,5)+I(2,2,5)-I(3,3,5)), m(5)*com(3,5);
              m(5)*com(1,5), m(5)*com(2,5), m(5)*com(3,5), m(5)];
   
   
    J(:,:,6)=[0.5*(-I(1,1,6)+I(2,2,6)+I(3,3,6)), I(1,2,6), I(1,3,6), m(6)*com(1,6);
             I(1,2,6) ,0.5*(I(1,1,6)-I(2,2,6)+I(3,3,6)), I(2,3,6), m(6)*com(2,6);
             I(1,3,6), I(2,3,6), 0.5*(I(1,1,6)+I(2,2,6)-I(3,3,6)), m(6)*com(3,6);
              m(6)*com(1,6), m(6)*com(2,6), m(6)*com(3,6), m(6)];
   
   
    J(:,:,7)=[0.5*(-I(1,1,7)+I(2,2,7)+I(3,3,7)), I(1,2,7), I(1,3,7), m(7)*com(1,7);
             I(1,2,7) ,0.5*(I(1,1,7)-I(2,2,7)+I(3,3,7)), I(2,3,7), m(7)*com(2,7);
             I(1,3,7), I(2,3,7), 0.5*(I(1,1,7)+I(2,2,7)-I(3,3,7)), m(7)*com(3,7);
              m(7)*com(1,7), m(7)*com(2,7), m(7)*com(3,7), m(7)];
   
   D=zeros(7,7);
    D(1,1)= trace(U(:,:,1,1)*J(:,:,1)*transpose(U(:,:,1,1))) + trace(U(:,:,2,1)*J(:,:,2)*transpose(U(:,:,2,1))) + trace(U(:,:,3,1)*J(:,:,3)*transpose(U(:,:,3,1))) + trace(U(:,:,4,1)*J(:,:,4)*transpose(U(:,:,4,1))) + trace(U(:,:,5,1)*J(:,:,5)*transpose(U(:,:,5,1))) + trace(U(:,:,6,1)*J(:,:,6)*transpose(U(:,:,6,1))) + trace(U(:,:,7,1)*J(:,:,7)*transpose(U(:,:,7,1))) ;
    D(1,2)= trace(U(:,:,2,2)*J(:,:,2)*transpose(U(:,:,2,1))) + trace(U(:,:,3,2)*J(:,:,3)*transpose(U(:,:,3,1))) + trace(U(:,:,4,2)*J(:,:,4)*transpose(U(:,:,4,1))) +trace(U(:,:,5,2)*J(:,:,5)*transpose(U(:,:,5,1))) + trace(U(:,:,6,2)*J(:,:,6)*transpose(U(:,:,6,1))) + trace(U(:,:,7,2)*J(:,:,7)*transpose(U(:,:,7,1))); 
    D(1,3)= trace(U(:,:,3,3)*J(:,:,3)*transpose(U(:,:,3,1)))+ trace(U(:,:,4,3)*J(:,:,4)*transpose(U(:,:,4,1)))+ trace(U(:,:,5,3)*J(:,:,5)*transpose(U(:,:,5,1)))+ trace(U(:,:,6,3)*J(:,:,6)*transpose(U(:,:,6,1)))+ trace(U(:,:,7,3)*J(:,:,7)*transpose(U(:,:,7,1))); 
    D(1,4)= trace(U(:,:,4,4)*J(:,:,4)*transpose(U(:,:,4,1)))+ trace(U(:,:,5,4)*J(:,:,5)*transpose(U(:,:,5,1)))+ trace(U(:,:,6,4)*J(:,:,6)*transpose(U(:,:,6,1)))+ trace(U(:,:,7,4)*J(:,:,7)*transpose(U(:,:,7,1)));
    D(1,5)= trace(U(:,:,5,5)*J(:,:,5)*transpose(U(:,:,5,1)))+ trace(U(:,:,6,5)*J(:,:,6)*transpose(U(:,:,6,1)))+ trace(U(:,:,7,5)*J(:,:,7)*transpose(U(:,:,7,1)));
    D(1,6)= trace(U(:,:,6,6)*J(:,:,6)*transpose(U(:,:,6,1)))+ trace(U(:,:,7,6)*J(:,:,7)*transpose(U(:,:,7,1)));
    D(1,7)= trace(U(:,:,7,7)*J(:,:,7)*transpose(U(:,:,7,1)));
    
    D(2,1)= trace(U(:,:,2,1)*J(:,:,2)*transpose(U(:,:,2,2)))+ trace(U(:,:,3,1)*J(:,:,3)*transpose(U(:,:,3,2)))+ trace(U(:,:,4,1)*J(:,:,4)*transpose(U(:,:,4,2)))+ trace(U(:,:,5,1)*J(:,:,5)*transpose(U(:,:,5,2)))+ trace(U(:,:,6,1)*J(:,:,6)*transpose(U(:,:,6,2)))+ trace(U(:,:,7,1)*J(:,:,7)*transpose(U(:,:,7,2)));
    D(2,2)= trace(U(:,:,2,2)*J(:,:,2)*transpose(U(:,:,2,2)))+ trace(U(:,:,3,2)*J(:,:,3)*transpose(U(:,:,3,2)))+ trace(U(:,:,4,2)*J(:,:,4)*transpose(U(:,:,4,2)))+ trace(U(:,:,5,2)*J(:,:,5)*transpose(U(:,:,5,2)))+ trace(U(:,:,6,2)*J(:,:,6)*transpose(U(:,:,6,2)))+ trace(U(:,:,7,2)*J(:,:,7)*transpose(U(:,:,7,2)));
    D(2,3)= trace(U(:,:,3,3)*J(:,:,3)*transpose(U(:,:,3,2)))+ trace(U(:,:,4,3)*J(:,:,4)*transpose(U(:,:,4,2)))+ trace(U(:,:,5,3)*J(:,:,5)*transpose(U(:,:,5,2)))+ trace(U(:,:,6,3)*J(:,:,6)*transpose(U(:,:,6,2)))+ trace(U(:,:,7,3)*J(:,:,7)*transpose(U(:,:,7,2))); 
    D(2,4)= trace(U(:,:,4,4)*J(:,:,4)*transpose(U(:,:,4,2)))+ trace(U(:,:,5,4)*J(:,:,5)*transpose(U(:,:,5,2)))+ trace(U(:,:,6,4)*J(:,:,6)*transpose(U(:,:,6,2)))+ trace(U(:,:,7,4)*J(:,:,7)*transpose(U(:,:,7,2))); 
    D(2,5)= trace(U(:,:,5,5)*J(:,:,5)*transpose(U(:,:,5,2)))+ trace(U(:,:,6,5)*J(:,:,6)*transpose(U(:,:,6,2)))+ trace(U(:,:,7,5)*J(:,:,7)*transpose(U(:,:,7,2)));
    D(2,6)= trace(U(:,:,6,6)*J(:,:,6)*transpose(U(:,:,6,2)))+ trace(U(:,:,7,6)*J(:,:,7)*transpose(U(:,:,7,2))); 
    D(2,7)= trace(U(:,:,7,7)*J(:,:,7)*transpose(U(:,:,7,2)));
  
    D(3,1)= trace(U(:,:,3,1)*J(:,:,3)*transpose(U(:,:,3,3)))+ trace(U(:,:,4,1)*J(:,:,4)*transpose(U(:,:,4,3)))+ trace(U(:,:,5,1)*J(:,:,5)*transpose(U(:,:,5,3)))+ trace(U(:,:,6,1)*J(:,:,6)*transpose(U(:,:,6,3)))+ trace(U(:,:,7,1)*J(:,:,7)*transpose(U(:,:,7,3)));
    D(3,2)= trace(U(:,:,3,2)*J(:,:,3)*transpose(U(:,:,3,3)))+ trace(U(:,:,4,2)*J(:,:,4)*transpose(U(:,:,4,3)))+ trace(U(:,:,5,2)*J(:,:,5)*transpose(U(:,:,5,3)))+ trace(U(:,:,6,2)*J(:,:,6)*transpose(U(:,:,6,3)))+ trace(U(:,:,7,2)*J(:,:,7)*transpose(U(:,:,7,3)));
    D(3,3)= trace(U(:,:,3,3)*J(:,:,3)*transpose(U(:,:,3,3)))+ trace(U(:,:,4,3)*J(:,:,4)*transpose(U(:,:,4,3)))+ trace(U(:,:,5,3)*J(:,:,5)*transpose(U(:,:,5,3)))+ trace(U(:,:,6,3)*J(:,:,6)*transpose(U(:,:,6,3)))+ trace(U(:,:,7,3)*J(:,:,7)*transpose(U(:,:,7,3)));
    D(3,4)= trace(U(:,:,4,4)*J(:,:,4)*transpose(U(:,:,4,3)))+ trace(U(:,:,5,4)*J(:,:,5)*transpose(U(:,:,5,3)))+ trace(U(:,:,6,4)*J(:,:,6)*transpose(U(:,:,6,3)))+ trace(U(:,:,7,4)*J(:,:,7)*transpose(U(:,:,7,3)));
    D(3,5)= trace(U(:,:,5,5)*J(:,:,5)*transpose(U(:,:,5,3)))+ trace(U(:,:,6,5)*J(:,:,6)*transpose(U(:,:,6,3)))+ trace(U(:,:,7,5)*J(:,:,7)*transpose(U(:,:,7,3)));
    D(3,6)= trace(U(:,:,6,6)*J(:,:,6)*transpose(U(:,:,6,3)))+ trace(U(:,:,7,6)*J(:,:,7)*transpose(U(:,:,7,3)));
    D(3,7)= trace(U(:,:,7,7)*J(:,:,7)*transpose(U(:,:,7,3)));
     
     
    D(4,1)= trace(U(:,:,4,1)*J(:,:,4)*transpose(U(:,:,4,4)))+ trace(U(:,:,5,1)*J(:,:,5)*transpose(U(:,:,5,4)))+ trace(U(:,:,6,1)*J(:,:,6)*transpose(U(:,:,6,4)))+ trace(U(:,:,7,1)*J(:,:,7)*transpose(U(:,:,7,4))); 
    D(4,2)= trace(U(:,:,4,2)*J(:,:,4)*transpose(U(:,:,4,4)))+ trace(U(:,:,5,2)*J(:,:,5)*transpose(U(:,:,5,4)))+ trace(U(:,:,6,2)*J(:,:,6)*transpose(U(:,:,6,4)))+ trace(U(:,:,7,2)*J(:,:,7)*transpose(U(:,:,7,4))); 
    D(4,3)= trace(U(:,:,4,3)*J(:,:,4)*transpose(U(:,:,4,4)))+ trace(U(:,:,5,3)*J(:,:,5)*transpose(U(:,:,5,4)))+ trace(U(:,:,6,3)*J(:,:,6)*transpose(U(:,:,6,4)))+ trace(U(:,:,7,3)*J(:,:,7)*transpose(U(:,:,7,4)));
    D(4,4)= trace(U(:,:,4,4)*J(:,:,4)*transpose(U(:,:,4,4)))+ trace(U(:,:,5,4)*J(:,:,5)*transpose(U(:,:,5,4)))+ trace(U(:,:,6,4)*J(:,:,6)*transpose(U(:,:,6,4)))+ trace(U(:,:,7,4)*J(:,:,7)*transpose(U(:,:,7,4)));
    D(4,5)= trace(U(:,:,5,5)*J(:,:,5)*transpose(U(:,:,5,4)))+ trace(U(:,:,6,5)*J(:,:,6)*transpose(U(:,:,6,4)))+ trace(U(:,:,7,5)*J(:,:,7)*transpose(U(:,:,7,4)));
    D(4,6)= trace(U(:,:,6,6)*J(:,:,6)*transpose(U(:,:,6,4)))+ trace(U(:,:,7,6)*J(:,:,7)*transpose(U(:,:,7,4))); 
    D(4,7)= trace(U(:,:,7,7)*J(:,:,7)*transpose(U(:,:,7,4)));
    
    D(5,1)= trace(U(:,:,5,1)*J(:,:,5)*transpose(U(:,:,5,5)))+ trace(U(:,:,6,1)*J(:,:,6)*transpose(U(:,:,6,5)))+ trace(U(:,:,7,1)*J(:,:,7)*transpose(U(:,:,7,5)));
    D(5,2)= trace(U(:,:,5,2)*J(:,:,5)*transpose(U(:,:,5,5)))+ trace(U(:,:,6,2)*J(:,:,6)*transpose(U(:,:,6,5)))+ trace(U(:,:,7,2)*J(:,:,7)*transpose(U(:,:,7,5)));
    D(5,3)= trace(U(:,:,5,3)*J(:,:,5)*transpose(U(:,:,5,5)))+ trace(U(:,:,6,3)*J(:,:,6)*transpose(U(:,:,6,5)))+ trace(U(:,:,7,3)*J(:,:,7)*transpose(U(:,:,7,5))); 
    D(5,4)= trace(U(:,:,5,4)*J(:,:,5)*transpose(U(:,:,5,5)))+ trace(U(:,:,6,4)*J(:,:,6)*transpose(U(:,:,6,5)))+ trace(U(:,:,7,4)*J(:,:,7)*transpose(U(:,:,7,5))); 
    D(5,5)= trace(U(:,:,5,5)*J(:,:,5)*transpose(U(:,:,5,5)))+ trace(U(:,:,6,5)*J(:,:,6)*transpose(U(:,:,6,5)))+ trace(U(:,:,7,5)*J(:,:,7)*transpose(U(:,:,7,5)));
    D(5,6)= trace(U(:,:,6,6)*J(:,:,6)*transpose(U(:,:,6,5)))+ trace(U(:,:,7,6)*J(:,:,7)*transpose(U(:,:,7,5))); 
    D(5,7)= trace(U(:,:,7,7)*J(:,:,7)*transpose(U(:,:,7,5)));
    
    D(6,1)= trace(U(:,:,6,1)*J(:,:,6)*transpose(U(:,:,6,6)))+ trace(U(:,:,7,1)*J(:,:,7)*transpose(U(:,:,7,6)));
    D(6,2)= trace(U(:,:,6,2)*J(:,:,6)*transpose(U(:,:,6,6)))+ trace(U(:,:,7,2)*J(:,:,7)*transpose(U(:,:,7,6)));
    D(6,3)= trace(U(:,:,6,3)*J(:,:,6)*transpose(U(:,:,6,6)))+ trace(U(:,:,7,3)*J(:,:,7)*transpose(U(:,:,7,6))); 
    D(6,4)= trace(U(:,:,6,4)*J(:,:,6)*transpose(U(:,:,6,6)))+ trace(U(:,:,7,4)*J(:,:,7)*transpose(U(:,:,7,6))); 
    D(6,5)= trace(U(:,:,6,5)*J(:,:,6)*transpose(U(:,:,6,6)))+ trace(U(:,:,7,5)*J(:,:,7)*transpose(U(:,:,7,6))); 
    D(6,6)= trace(U(:,:,6,6)*J(:,:,6)*transpose(U(:,:,6,6)))+ trace(U(:,:,7,6)*J(:,:,7)*transpose(U(:,:,7,6))); 
    D(6,7)= trace(U(:,:,7,7)*J(:,:,7)*transpose(U(:,:,7,6)));
    
    D(7,1)= trace(U(:,:,7,1)*J(:,:,7)*transpose(U(:,:,7,7)));
    D(7,2)= trace(U(:,:,7,2)*J(:,:,7)*transpose(U(:,:,7,7)));
    D(7,3)= trace(U(:,:,7,3)*J(:,:,7)*transpose(U(:,:,7,7)));
    D(7,4)= trace(U(:,:,7,4)*J(:,:,7)*transpose(U(:,:,7,7)));
    D(7,5)= trace(U(:,:,7,5)*J(:,:,7)*transpose(U(:,:,7,7)));
    D(7,6)= trace(U(:,:,7,6)*J(:,:,7)*transpose(U(:,:,7,7)));
    D(7,7)= trace(U(:,:,7,7)*J(:,:,7)*transpose(U(:,:,7,7)));
end 



function T = getTransformDH(a,d,alpha,q)
    ct = cos(q);
    st = sin(q);
    cb = cos(alpha);
    sb = sin(alpha);
    
    T = [ ct, -st*cb,  st*sb, a*ct;
          st,  ct*cb, -ct*sb, a*st;
          0, sb, cb, d;
          0, 0, 0, 1 ];
end
